simulink model "Part3_newest"  (R2017a)
settings: Solver=VariableStepAuto  StartTime=0.0  StopTime=0.1  RelTol=1e-3
libraries: commdigbbndam3 x2, commchan3 x1, commsink2 x1, commrandsrc2 x1
settings Model: Creator=Marine  LastModifiedBy=mhuynh7
settings SFSimCC: SimUseLocalCustomCode=on
settings RTWCC: RTWUseLocalCustomCode=on

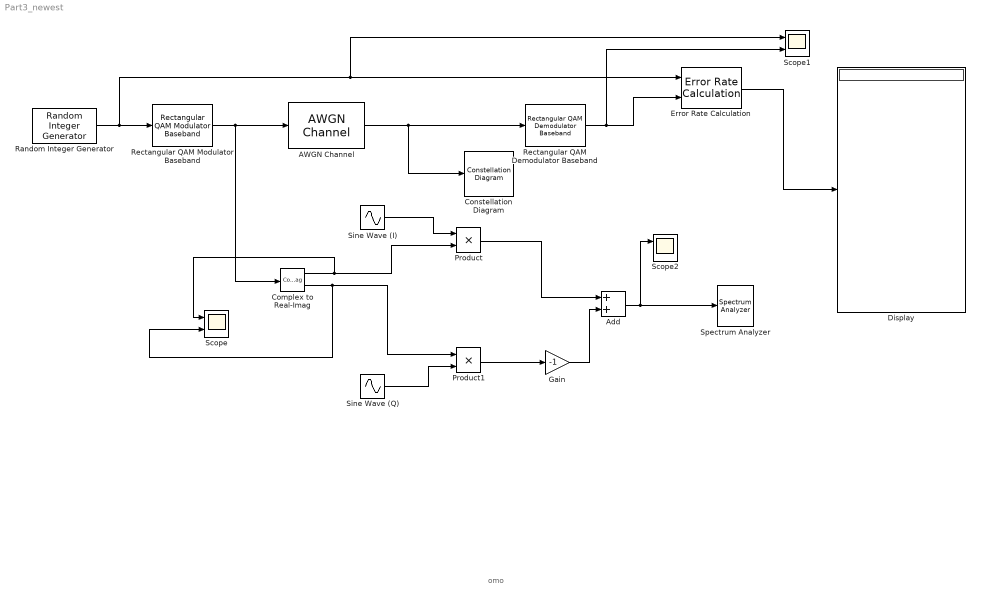
== system Part3_newest ==
  note: omo
  AWGN Channel : commchan3/AWGN Channel  InputProcessing=Columns as channels (frame based)  seed=randseed  noiseMode="Signal to noise ratio  (Eb/No)"  EbNodB=0  EsNodB=10  SNRdB=10  bitsPerSym=4  Ps=1  Tsym=1e-3  variance=1
  Add : Sum
  Complex to Real-Imag : ComplexToRealImag
  Constellation Diagram : ConstellationDiagram
  Display : Display
  Error Rate Calculation : commsink2/Error Rate Calculation  N=0  st_delay=0  cp_mode=Entire frame  subframe=[]  PMode=Port  WsName=ErrorVec  RsMode2=off  stop=on  numErr=100  maxBits=1e6
  Gain : Gain  Gain=-1
  Product : Product
  Product1 : Product
  Random Integer Generator : commrandsrc2/Random Integer Generator  mul=16  seed=randseed  Ts=1e-3  frameBased=on  sampPerFrame=2500  orient=off  outDataType=double
  Rectangular QAM Demodulator Baseband : commdigbbndam3/Rectangular QAM Demodulator Baseband  M=16  OutType=Integer  DecType=Hard decision  VarSource=Dialog  Variance=1  Dec=Gray  Mapping=[0:15]  PowType=Average Power  MinDist=2  AvgPow=1  PeakPow=1  Ph=0  outDtype1=Inherit via internal rule  outDtype2=Inherit via internal rule  derotateFactorWordLen=16  derotateFactorDataTypeStr=Inherit: Same word length as input  derotateFactorLastDataTypeStr=Inherit: Same word length as input  denormFactorWordLen=16  denormFactorDataTypeStr=Inherit: Same word length as input  denormFactorLastDataTypeStr=Inherit: Same word length as input  prodOutWordLen=32  prodOutOverflowMode=Wrap  prodOutRoundingMode=Floor  prodOutOvFlMode=off  prodOutOvFlModeLastStrValue=off  sumWordLen=32
  Rectangular QAM Modulator Baseband : commdigbbndam3/Rectangular QAM Modulator Baseband  M=16  InType=Integer  Enc=Gray  Mapping=[0:15]  PowType=Average Power  MinDist=2  AvgPow=1  PeakPow=1  Ph=0  outDtype=double  outWordLen=16  outUDDataType=sfix(16)  outFracLenMode=Best precision  outFracLen=15  outDataTypeStr=double  outLastDataTypeStr=double
  Scope : Scope  NumInputPorts=2
  Scope1 : Scope  NumInputPorts=2
  Scope2 : Scope  NumInputPorts=2
  Sine Wave (I) : Sin  Frequency=1e4  Phase=pi/2  SampleTime=1e-6
  Sine Wave (Q) : Sin  Frequency=1e4  SampleTime=1e-6
  Spectrum Analyzer : SpectrumAnalyzer
  wires:
  Complex to Real-Imag/2 -> Scope/2, Product1/1
  Sine Wave (Q)/1 -> Product1/2
  Complex to Real-Imag/1 -> Scope/1, Product/2
  Sine Wave (I)/1 -> Product/1
  Product1/1 -> Gain/1
  Gain/1 -> Add/2
  Product/1 -> Add/1
  Add/1 -> Scope2/1, Spectrum Analyzer/1
  Random Integer Generator/1 -> Scope1/1, Error Rate Calculation/1, Rectangular QAM Modulator Baseband/1
  Rectangular QAM Modulator Baseband/1 -> Complex to Real-Imag/1, AWGN Channel/1
  AWGN Channel/1 -> Constellation Diagram/1, Rectangular QAM Demodulator Baseband/1
  Rectangular QAM Demodulator Baseband/1 -> Scope1/2, Error Rate Calculation/2
  Error Rate Calculation/1 -> Display/1
